simulink model "tpSimul"  (R2019b)
settings: Solver=VariableStepAuto  StartTime=0.0  StopTime=12  RelTol=1e-3
values from neighbouring files (symbols this model uses):
  A = [0 (M+m)*g/(M*l) 0 0;1 0 0 0;0 -m*g/M 0 0;0 0 1 0]    [TP.m]
  B = [-1/(M*l); 0; 1/M; 0]    [TP.m]
  C = [0 0 0 1]    [TP.m]
  calGain = 1/dcgain(cltf)    [TP.m]
  K = acker(A,B,phi)    [TP.m]
settings Model: Creator=m214134  LastModifiedBy=m214134

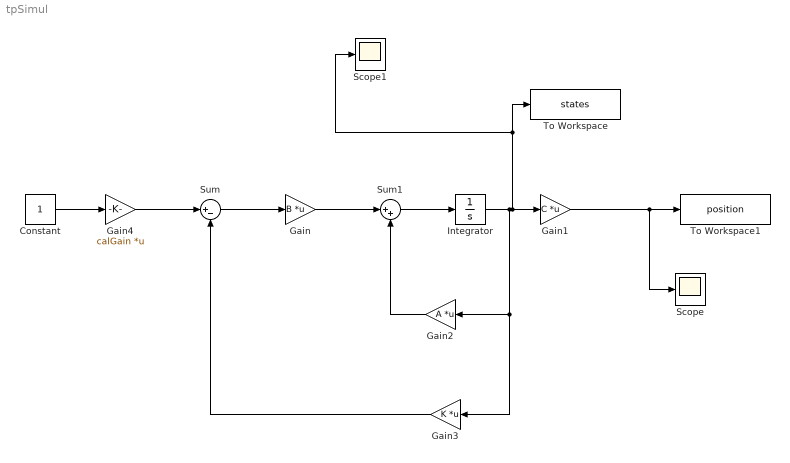
== system tpSimul ==
  Constant : Constant
  Gain : Gain  Gain=B  Multiplication=Matrix(K*u)
  Gain1 : Gain  Gain=C  Multiplication=Matrix(K*u)
  Gain2 : Gain  Gain=A  Multiplication=Matrix(K*u)
  Gain3 : Gain  Gain=K  Multiplication=Matrix(K*u)
  Gain4 : Gain  Gain=calGain  Multiplication=Matrix(K*u)
  Integrator : Integrator
  Scope : Scope
  Scope1 : Scope
  Sum : Sum  Inputs=|+-
  Sum1 : Sum  Inputs=|++
  To Workspace : ToWorkspace  VariableName=states  SaveFormat=Timeseries  SampleTime=-1
  To Workspace1 : ToWorkspace  VariableName=position  SaveFormat=Timeseries  SampleTime=-1
  wires:
  Integrator/1 -> Gain3/1, Gain2/1, Scope1/1, To Workspace/1, Gain1/1
  Gain1/1 -> Scope/1, To Workspace1/1
  Sum/1 -> Gain/1
  Sum1/1 -> Integrator/1
  Gain/1 -> Sum1/1
  Constant/1 -> Gain4/1
  Gain2/1 -> Sum1/2
  Gain3/1 -> Sum/2
  Gain4/1 -> Sum/1
